simulink model "RoboBoat_Circle_SLAM_v1"  (R2014a)
settings: Solver=FixedStepDiscrete  StartTime=0.0  StopTime=inf  FixedStep=.1  RelTol=1e-3
undefined symbols (not defined in the file): Com1, Com2, Com3, Com4, DiscIntNeverNeededParam, standard
libraries: xpcseriallib x29, slrtlib x5, speedgoatlib_IO102 x5, speedgoatlib x1
(part 1 of 2)
settings Model: BufferReuse=off  Creator=wildcat  LastModifiedBy=wildcat
settings SolverCC: EnableConcurrentExecution=on
settings DataIOCC: SignalLoggingSaveFormat=ModelDataLogs
settings OptimizationCC: BlockReduction=off  OptimizeBlockIOStorage=off  BufferReuse=off  GlobalBufferReuse=off  ExpressionFolding=off  LocalBlockOutputs=off
settings DebuggingCC: UnderspecifiedInitializationDetection=Classic  MultiTaskDSMMsg=warning  StateNameClashWarn=warning
settings HardwareCC: ProdIntDivRoundTo=Zero  ProdEndianess=LittleEndian  ProdHWDeviceType=Generic->32-bit x86 compatible
settings RTWCC: SystemTargetFile=slrt.tlc  TemplateMakefile=slrt_default_tmf  Description=Simulink Real-Time  ProcessScript=slrt_make_rtw_hook  RTWCompilerOptimization=On
settings SimulinkRealTimeCC: GeneratePreprocessorConditionals=Disable all  EnableShiftOperators=on

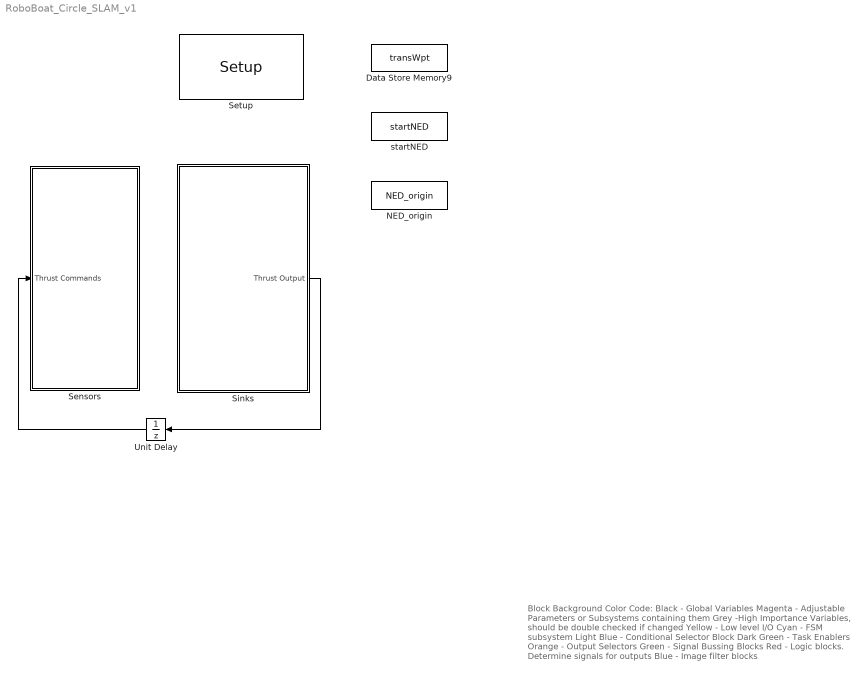
== system RoboBoat_Circle_SLAM_v1 ==
  note: Block Background Color Code:
      | Black - Global Variables
      | Magenta - Adjustable Parameters or Subsystems containing them
      | Grey -High Importance Variables, should be double checked if changed
      | Yellow - Low level I/O
      | Cyan - FSM subsystem
      | Light Blue - Conditional Selector Block
      | Dark Green - Task Enablers
      | Orange - Output Selectors
      | Green - Signal Bussing Blocks
      | Red - Logic blocks. Determine signals for outputs
      | Blue - Image filter blocks
  Data Store Memory9 : DataStoreMemory  DataStoreName=transWpt  ReadBeforeWriteMsg=warning  WriteAfterWriteMsg=warning  WriteAfterReadMsg=warning  InitialValue=[4009.4964500000, 7532.95009000000]
  NED_origin : DataStoreMemory  DataStoreName=NED_origin  ReadBeforeWriteMsg=warning  WriteAfterWriteMsg=warning  WriteAfterReadMsg=warning  InitialValue=[40.1584510000000, -75.5492320000000]  VectorParams1D=off
  Sensors : Subsystem
  Setup : speedgoatlib_IO102/Setup  group=Analog input setup  id=1  range=+-5V  cal=off  pciSlot=-1  adChannelMode=Multiple-channel (enter number of channels below)  adChannel=16  adCoupling=Differential  daChannel=[1,2,3,4]  daReset=[1]  daInitValue=[0]  diChannel=[1,2,3,4,5,6,7,8]  doChannel=[1,2,3,4,5,6,7,8]  doReset=[1]  doInitValue=[0]
  Sinks : Subsystem
  Unit Delay : UnitDelay  SampleTime=-1
  startNED : DataStoreMemory  DataStoreName=startNED  ReadBeforeWriteMsg=warning  WriteAfterWriteMsg=warning  WriteAfterReadMsg=warning  InitialValue=[-10.1298988348139, -7.82721042881905]  VectorParams1D=off
  wires:
  Sinks/1(Thrust Output) -> Unit Delay/1
  Unit Delay/1 -> Sensors/1(Thrust Commands)

== system RoboBoat_Circle_SLAM_v1/Sensors ==
  Thrust Commands : Inport
  1020 Comms : Subsystem  Commented=on
  Baseboard Serial : Subsystem
  Bus Creator : BusCreator  Inputs=3
  IO102 : Subsystem
  data log : Subsystem
  wires:
  Baseboard Serial/1(Serial Inputs) -> Bus Creator/1
  Bus Creator/1 -> data log/1(Sensors signal)  "Serial In"
  IO102/1(IO102 Inputs) -> Bus Creator/2
  Thrust Commands/1 -> Bus Creator/3  "Thrust"

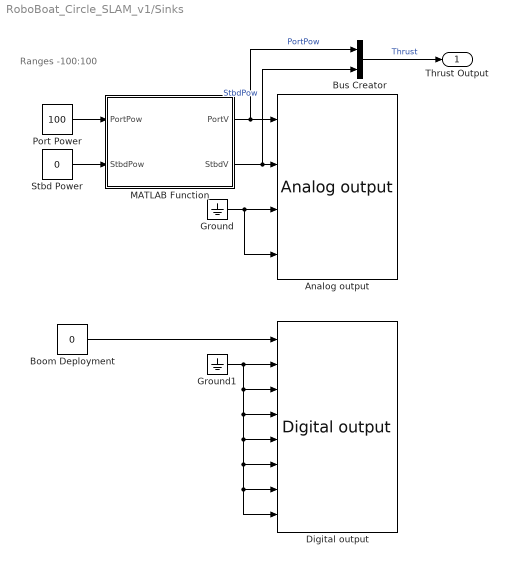
== system RoboBoat_Circle_SLAM_v1/Sinks ==
  note: Ranges -100:100
  Analog output : speedgoatlib_IO102/Analog output  id=1  channels=[1,2,3,4]  range=2  ts=-1  pciSlot=-1
  Boom Deployment : Constant  Value=0
  Bus Creator : BusCreator  Inputs=2
  Digital output : speedgoatlib_IO102/Digital output  id=1  channels=[1,2,3,4,5,6,7,8]  ts=-1  pciSlot=-1
  Ground : Ground
  Ground1 : Ground
  MATLAB Function : MATLAB Function  TreatAsAtomicUnit=on
  Port Power : Constant  Value=100
  Stbd Power : Constant  Value=0
  Thrust Output : Outport
  wires:
  Ground/1 -> Analog output/4, Analog output/3
  Port Power/1 -> MATLAB Function/1(PortPow)
  Stbd Power/1 -> MATLAB Function/2(StbdPow)
  Boom Deployment/1 -> Digital output/1
  Ground1/1 -> Digital output/3, Digital output/4, Digital output/5, Digital output/6, Digital output/7, Digital output/8, Digital output/2
  MATLAB Function/1(PortV) -> Bus Creator/1, Analog output/1  "PortPow"
  MATLAB Function/2(StbdV) -> Bus Creator/2, Analog output/2  "StbdPow"
  Bus Creator/1 -> Thrust Output/1  "Thrust"

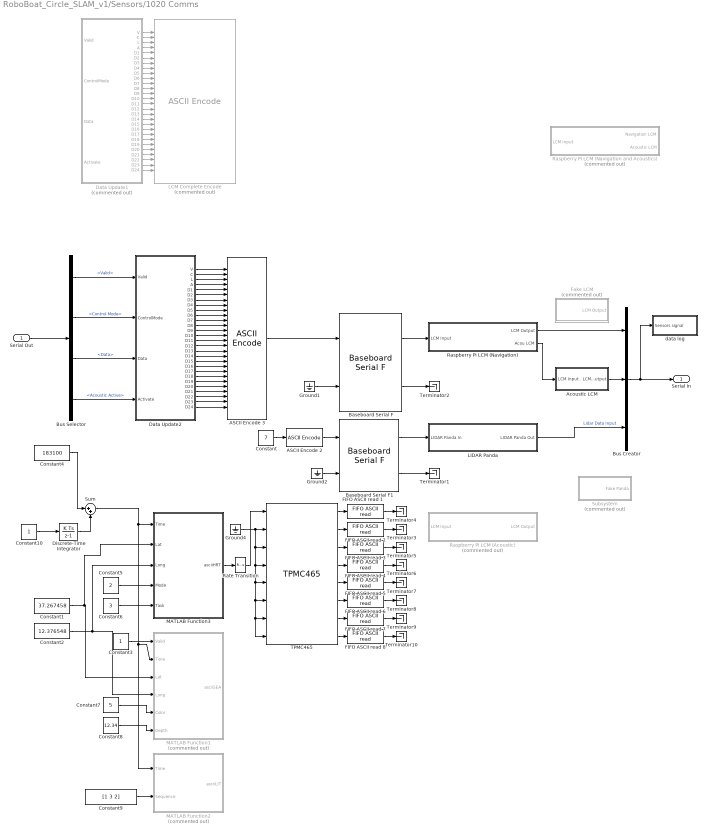
== system RoboBoat_Circle_SLAM_v1/Sensors/1020 Comms ==
  Serial Out : Inport
  " Raspberry Pi LCM (Acoustic)" : Subsystem  Commented=on
  " Raspberry Pi LCM (Navigation and Acoustics)" : Subsystem  Commented=on
  " Raspberry Pi LCM (Navigation)" : Subsystem
  ASCII Encode 2 : xpcseriallib/ASCII Encode   format=SGTask:%d \r\n  nvars=1  maxlength=128  vartypes={ 'double' }
  ASCII Encode 3 : xpcseriallib/ASCII Encode   format="{\"Valid\":%d, \"Mode\":%d, \"Length\":%d, \"Activate\":%d, \"Waypoints\":[%f, %f, %f, %f, %f, %f, %f, %f, %f, %f, %f, %f, %f, %f, %f, %f, %f, %f, %f, %f, %f, %f, %f, %f]} \\r\\n"  nvars=28  maxlength=1000  vartypes={ 'double' }
  Acoustic LCM : Subsystem
  Baseboard Serial F : xpcseriallib/Mainboard/Baseboard Serial F  group=Basic Setup  port=1  irqnum=4  saddr1=0x3f8  saddr2=0x3e8  config=Com1/Com3  baud1=115200  parity1=Even  ndata1=7  nstop1=1  fifomode1=64 deep  rlevel1=1  automode1=on  xmtfifosize1=1024  xmtdatatype1=8 bit uint null terminated  rcvfifosize1=1024  baud2=115200  parity2=Even  ndata2=7  nstop2=1  fifomode2=64 deep  rlevel2=1  automode2=on  xmtfifosize2=1024  xmtdatatype2=8 bit uint null terminated  rcvfifosize2=1024
  Baseboard Serial F1 : xpcseriallib/Mainboard/Baseboard Serial F  group=FIFO Setup  port=1  irqnum=4  saddr1=0x3f8  saddr2=0x3e8  config=Com2/Com4  baud1=115200  parity1=Even  ndata1=7  nstop1=1  fifomode1=64 deep  rlevel1=1  automode1=on  xmtfifosize1=1024  xmtdatatype1=8 bit uint null terminated  rcvfifosize1=1024  baud2=115200  parity2=Even  ndata2=7  nstop2=1  fifomode2=64 deep  rlevel2=1  automode2=on  xmtfifosize2=1024  xmtdatatype2=8 bit uint null terminated  rcvfifosize2=1024
  Bus Creator : BusCreator  Inputs=3
  Bus Selector : BusSelector  OutputSignals=Outputs.Navigation Outputs.Valid,Outputs.Navigation Outputs.Control Mode,Outputs.Navigation Outputs.Data,Outputs.Acoustic Active
  Constant : Constant  Value=7
  Constant1 : Constant  Value=37.267458
  Constant10 : Constant
  Constant2 : Constant  Value=12.376548
  Constant3 : Constant
  Constant4 : Constant  Value=183100
  Constant5 : Constant  Value=2
  Constant6 : Constant  Value=3
  Constant7 : Constant  Value=5
  Constant8 : Constant  Value=12.34
  Constant9 : Constant  Value=[1 3 2]
  Data Update1 : MATLAB Function  Commented=on  TreatAsAtomicUnit=on
  Data Update2 : MATLAB Function  TreatAsAtomicUnit=on
  Discrete-Time Integrator : DiscreteIntegrator  SampleTime=-1  ICPrevOutput=DiscIntNeverNeededParam  ICPrevScaledInput=DiscIntNeverNeededParam
  FIFO ASCII read {1..8} (8 alike) : xpcseriallib/FIFO ASCII read   header={'Deploy:'}  term=[13 10]  hold=Zero output if no new data  enable=off  maxsize=1024  outputtype=8 bit uint null terminated  sampletime=-1
  Fake LCM : Subsystem  Commented=on
  Ground1 : Ground
  Ground2 : Ground
  Ground4 : Ground
  LCM Complete Encode : xpcseriallib/ASCII Encode   Commented=on  format="{\"Valid\":%d, \"Mode\":%d, \"Length\":%d, \"Activate\":%d, \"Waypoints\":[%f, %f, %f, %f, %f, %f, %f, %f, %f, %f, %f, %f, %f, %f, %f, %f, %f, %f, %f, %f, %f, %f, %f, %f]} \\r\\n"  nvars=28  maxlength=1000  vartypes={ 'double' }
  LIDAR Panda : Subsystem
  MATLAB Function1 : MATLAB Function  Commented=on  TreatAsAtomicUnit=on
  MATLAB Function2 : MATLAB Function  Commented=on  TreatAsAtomicUnit=on
  MATLAB Function3 : MATLAB Function  TreatAsAtomicUnit=on
  Rate Transition : RateTransition  Deterministic=off  OutPortSampleTime=1
  Subsystem : Subsystem  Commented=on
  Sum : Sum  Inputs=|++
  TPMC465 : speedgoatlib/IO504/TPMC465  group=Basic Setup  port=2  irqnum=9  slot=-1  transceiver1=RS232 (max 921.6kb/s)  standard1=on  baud1=115200  bauddivisor1=1  sampling1=16x (standard)  prescale1=off  parity1=Even  ndata1=7  nstop1=1  rlevel1=half full (32)  hwmode1=none  swmode1=none  xonchar1=17  xoffchar1=19  rs485auto1=off  rs485delay1=0  xmtfifosize1=1024  xmtdatatype1=8 bit uint null terminated  rcvfifosize1=1024  transceiver2=RS232 (max 921.6kb/s)  standard2=on  baud2=115200  bauddivisor2=1  sampling2=16x (standard)  prescale2=off  parity2=Even  ndata2=7  nstop2=1  rlevel2=half full (32)  hwmode2=none  swmode2=none  xonchar2=17  xoffchar2=19  rs485auto2=off  rs485delay2=0  xmtfifosize2=1024  xmtdatatype2=8 bit uint null terminated  rcvfifosize2=1024  transceiver3=RS232 (max 921.6kb/s)  standard3=on  baud3=115200  bauddivisor3=1  sampling3=16x (standard)  prescale3=off  parity3=Even  ndata3=7  nstop3=1  rlevel3=half full (32)  hwmode3=none  swmode3=none  xonchar3=17  xoffchar3=19  rs485auto3=off  rs485delay3=0  xmtfifosize3=1024  xmtdatatype3=8 bit uint null terminated  rcvfifosize3=1024  transceiver4=RS232 (max 921.6kb/s)  standard4=on  baud4=115200  bauddivisor4=1  sampling4=16x (standard)  prescale4=off  parity4=None  ndata4=8  nstop4=1  rlevel4=half full (32)  hwmode4=none  swmode4=none  xonchar4=17  xoffchar4=19  rs485auto4=off  rs485delay4=0  xmtfifosize4=1024  xmtdatatype4=8 bit uint null terminated  rcvfifosize4=1024  transceiver5=RS232 (max 921.6kb/s)  standard5=on  baud5=115200  bauddivisor5=1  sampling5=16x (standard)  prescale5=off  parity5=None  ndata5=8  nstop5=1  rlevel5=1  hwmode5=none  swmode5=none  xonchar5=17  xoffchar5=19  rs485auto5=off  rs485delay5=0  xmtfifosize5=1024  xmtdatatype5=8 bit uint null terminated  rcvfifosize5=1024  transceiver6=RS232 (max 921.6kb/s)  standard6=on  baud6=115200  bauddivisor6=1  sampling6=16x (standard)  prescale6=off  parity6=None  ndata6=8  nstop6=1  rlevel6=1  hwmode6=none  swmode6=none  xonchar6=17  xoffchar6=19  rs485auto6=off  rs485delay6=0  xmtfifosize6=1024  xmtdatatype6=8 bit uint null terminated  rcvfifosize6=1024  transceiver7=RS232 (max 921.6kb/s)  standard7=on  baud7=115200  bauddivisor7=1  sampling7=16x (standard)  prescale7=off  parity7=None  ndata7=8  nstop7=1  rlevel7=1  hwmode7=none  swmode7=none  xonchar7=17  xoffchar7=19  rs485auto7=off  rs485delay7=0  xmtfifosize7=1024  xmtdatatype7=8 bit uint null terminated  rcvfifosize7=1024  transceiver8=RS232 (max 921.6kb/s)  standard8=on  baud8=115200  bauddivisor8=1  sampling8=16x (standard)  prescale8=off  parity8=None  ndata8=8  nstop8=1  rlevel8=1  hwmode8=none  swmode8=none  xonchar8=17  xoffchar8=19  rs485auto8=off  rs485delay8=0  xmtfifosize8=1024  xmtdatatype8=8 bit uint null terminated  rcvfifosize8=1024
  Terminator{1..10} (10 alike) : Terminator
  data log : Subsystem
  Serial In : Outport
  wires:
  Serial Out/1 -> Bus Selector/1
  Baseboard Serial F/1 -> " Raspberry Pi LCM (Navigation)"/1(LCM Input)
  ASCII Encode 3/1 -> Baseboard Serial F/1
  " Raspberry Pi LCM (Navigation)"/1(LCM Output) -> Bus Creator/1
  Bus Selector/1 -> Data Update2/1(Valid)  "<Valid>"
  Bus Selector/2 -> Data Update2/2(ControlMode)  "<Control Mode>"
  Bus Selector/3 -> Data Update2/3(Data)  "<Data>"
  Acoustic LCM/1(LCM Output) -> Bus Creator/2
  Baseboard Serial F/2 -> Terminator2/1
  Ground1/1 -> Baseboard Serial F/2
  LIDAR Panda/1(LIDAR Panda Out) -> Bus Creator/3  "Lidar Data Input"
  Bus Creator/1 -> Serial In/1, data log/1(Sensors signal)
  Data Update1/1(V) -> LCM Complete Encode/1
  Data Update1/2(C) -> LCM Complete Encode/2
  Data Update1/6(D2) -> LCM Complete Encode/6
  Data Update1/7(D3) -> LCM Complete Encode/7
  Data Update1/8(D4) -> LCM Complete Encode/8
  Data Update1/5(D1) -> LCM Complete Encode/5
  Data Update1/9(D5) -> LCM Complete Encode/9
  Data Update1/10(D6) -> LCM Complete Encode/10
  Data Update1/11(D7) -> LCM Complete Encode/11
  Data Update1/12(D8) -> LCM Complete Encode/12
  Data Update1/13(D9) -> LCM Complete Encode/13
  Data Update1/18(D14) -> LCM Complete Encode/18
  Data Update1/15(D11) -> LCM Complete Encode/15
  Data Update1/20(D16) -> LCM Complete Encode/20
  Data Update1/21(D17) -> LCM Complete Encode/21
  Data Update1/19(D15) -> LCM Complete Encode/19
  Data Update1/14(D10) -> LCM Complete Encode/14
  Data Update1/16(D12) -> LCM Complete Encode/16
  Data Update1/22(D18) -> LCM Complete Encode/22
  Data Update1/23(D19) -> LCM Complete Encode/23
  Data Update1/24(D20) -> LCM Complete Encode/24
  Data Update1/25(D21) -> LCM Complete Encode/25
  Data Update1/27(D23) -> LCM Complete Encode/27
  Data Update1/26(D22) -> LCM Complete Encode/26
  Data Update1/28(D24) -> LCM Complete Encode/28
  Data Update1/3(L) -> LCM Complete Encode/3
  Data Update1/4(A) -> LCM Complete Encode/4
  Data Update1/17(D13) -> LCM Complete Encode/17
  " Raspberry Pi LCM (Navigation)"/2(Acou LCM) -> Acoustic LCM/1(LCM Input)
  Data Update2/21(D17) -> ASCII Encode 3/21
  Data Update2/20(D16) -> ASCII Encode 3/20
  Data Update2/19(D15) -> ASCII Encode 3/19
  Data Update2/4(A) -> ASCII Encode 3/4
  Data Update2/2(C) -> ASCII Encode 3/2
  Data Update2/18(D14) -> ASCII Encode 3/18
  Data Update2/16(D12) -> ASCII Encode 3/16
  Data Update2/7(D3) -> ASCII Encode 3/7
  Data Update2/6(D2) -> ASCII Encode 3/6
  Data Update2/5(D1) -> ASCII Encode 3/5
  Data Update2/17(D13) -> ASCII Encode 3/17
  Data Update2/9(D5) -> ASCII Encode 3/9
  Data Update2/10(D6) -> ASCII Encode 3/10
  Data Update2/24(D20) -> ASCII Encode 3/24
  Data Update2/23(D19) -> ASCII Encode 3/23
  Data Update2/28(D24) -> ASCII Encode 3/28
  Data Update2/26(D22) -> ASCII Encode 3/26
  Data Update2/25(D21) -> ASCII Encode 3/25
  Data Update2/3(L) -> ASCII Encode 3/3
  Data Update2/27(D23) -> ASCII Encode 3/27
  Data Update2/8(D4) -> ASCII Encode 3/8
  Data Update2/11(D7) -> ASCII Encode 3/11
  Data Update2/13(D9) -> ASCII Encode 3/13
  Data Update2/12(D8) -> ASCII Encode 3/12
  Data Update2/14(D10) -> ASCII Encode 3/14
  Data Update2/22(D18) -> ASCII Encode 3/22
  Data Update2/15(D11) -> ASCII Encode 3/15
  Bus Selector/4 -> Data Update2/4(Activate)  "<Acoustic Active>"
  Data Update2/1(V) -> ASCII Encode 3/1
  Constant9/1 -> MATLAB Function2/2(Sequence)
  Constant7/1 -> MATLAB Function1/5(Color)
  Constant8/1 -> MATLAB Function1/6(Depth)
  Constant5/1 -> MATLAB Function3/4(Mode)
  Constant6/1 -> MATLAB Function3/5(Task)
  Sum/1 -> MATLAB Function3/1(Time), MATLAB Function2/1(Time), MATLAB Function1/2(Time)
  Constant2/1 -> MATLAB Function3/3(Long), MATLAB Function1/4(Long)
  Constant1/1 -> MATLAB Function3/2(Lat), MATLAB Function1/3(Lat)
  Ground4/1 -> TPMC465/2, TPMC465/3, TPMC465/4, TPMC465/8, TPMC465/7, TPMC465/6, TPMC465/5
  TPMC465/1 -> FIFO ASCII read 1/1
  FIFO ASCII read 1/1 -> Terminator4/1
  FIFO ASCII read 2/1 -> Terminator3/1
  FIFO ASCII read 3/1 -> Terminator5/1
  FIFO ASCII read 4/1 -> Terminator6/1
  FIFO ASCII read 5/1 -> Terminator7/1
  FIFO ASCII read 6/1 -> Terminator8/1
  FIFO ASCII read 7/1 -> Terminator9/1
  FIFO ASCII read 8/1 -> Terminator10/1
  TPMC465/2 -> FIFO ASCII read 2/1
  TPMC465/3 -> FIFO ASCII read 3/1
  TPMC465/4 -> FIFO ASCII read 4/1
  TPMC465/5 -> FIFO ASCII read 5/1
  TPMC465/6 -> FIFO ASCII read 6/1
  TPMC465/7 -> FIFO ASCII read 7/1
  TPMC465/8 -> FIFO ASCII read 8/1
  Rate Transition/1 -> TPMC465/1
  Constant3/1 -> MATLAB Function1/1(Valid)
  MATLAB Function3/1(asciiHRT) -> Rate Transition/1
  Constant4/1 -> Sum/1
  Discrete-Time Integrator/1 -> Sum/2
  Constant10/1 -> Discrete-Time Integrator/1
  Baseboard Serial F1/1 -> LIDAR Panda/1(LIDAR Panda In)
  Ground2/1 -> Baseboard Serial F1/2
  Baseboard Serial F1/2 -> Terminator1/1
  ASCII Encode 2/1 -> Baseboard Serial F1/1
  Constant/1 -> ASCII Encode 2/1

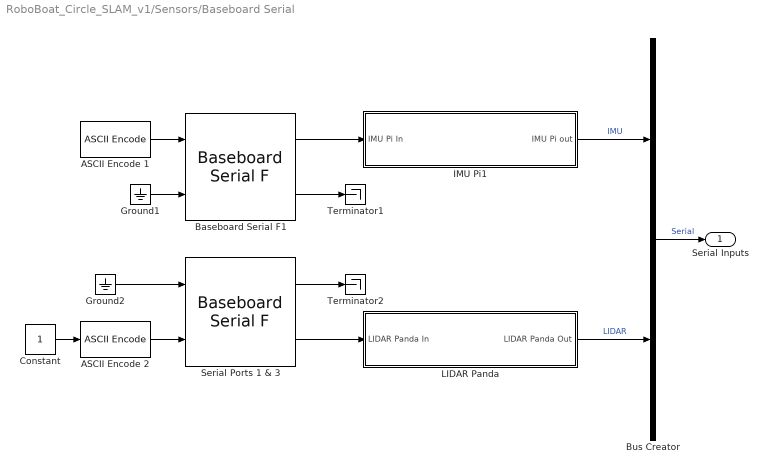
== system RoboBoat_Circle_SLAM_v1/Sensors/Baseboard Serial ==
  ASCII Encode 1 : xpcseriallib/ASCII Encode   format=SGB \r\n  nvars=0  maxlength=128  vartypes={ 'double' }
  ASCII Encode 2 : xpcseriallib/ASCII Encode   format=SGTask:%d \r\n  nvars=1  maxlength=128  vartypes={ 'double' }
  Baseboard Serial F1 : xpcseriallib/Mainboard/Baseboard Serial F  group=Basic Setup  port=1  irqnum=4  saddr1=0x3f8  saddr2=0x3e8  config=Com2/Com4  baud1=115200  parity1=Even  ndata1=7  nstop1=1  fifomode1=64 deep  rlevel1=1  automode1=on  xmtfifosize1=1024  xmtdatatype1=8 bit uint null terminated  rcvfifosize1=1024  baud2=115200  parity2=Even  ndata2=7  nstop2=1  fifomode2=64 deep  rlevel2=1  automode2=on  xmtfifosize2=1024  xmtdatatype2=8 bit uint null terminated  rcvfifosize2=1024
  Bus Creator : BusCreator  Inputs=2
  Constant : Constant
  Ground1 : Ground
  Ground2 : Ground
  IMU Pi1 : Subsystem
  LIDAR Panda : Subsystem
  Serial Ports 1 & 3 : xpcseriallib/Mainboard/Baseboard Serial F  group=Basic Setup  port=2  irqnum=4  saddr1=0x3f8  saddr2=0x3e8  config=Com1/Com3  baud1=115200  parity1=Even  ndata1=7  nstop1=1  fifomode1=64 deep  rlevel1=1  automode1=on  xmtfifosize1=1024  xmtdatatype1=8 bit uint null terminated  rcvfifosize1=1024  baud2=115200  parity2=Even  ndata2=7  nstop2=1  fifomode2=64 deep  rlevel2=1  automode2=on  xmtfifosize2=1024  xmtdatatype2=8 bit uint null terminated  rcvfifosize2=1024
  Terminator1 : Terminator
  Terminator2 : Terminator
  Serial Inputs : Outport
  wires:
  Baseboard Serial F1/1 -> IMU Pi1/1(IMU Pi In)
  Ground1/1 -> Baseboard Serial F1/2
  Baseboard Serial F1/2 -> Terminator1/1
  Ground2/1 -> Serial Ports 1 & 3/1
  Serial Ports 1 & 3/2 -> LIDAR Panda/1(LIDAR Panda In)
  Constant/1 -> ASCII Encode 2/1
  ASCII Encode 2/1 -> Serial Ports 1 & 3/2
  Serial Ports 1 & 3/1 -> Terminator2/1
  LIDAR Panda/1(LIDAR Panda Out) -> Bus Creator/2  "LIDAR"
  Bus Creator/1 -> Serial Inputs/1  "Serial"
  IMU Pi1/1(IMU Pi out) -> Bus Creator/1  "IMU"
  ASCII Encode 1/1 -> Baseboard Serial F1/1

== system RoboBoat_Circle_SLAM_v1/Sensors/IO102 ==
  Analog In : Subsystem
  Bus Creator : BusCreator  Inputs=2
  Digital In : Subsystem
  IO102 Inputs : Outport
  wires:
  Digital In/1(Digital In) -> Bus Creator/1  "Digital"
  Analog In/1(Analog In) -> Bus Creator/2  "Analog"
  Bus Creator/1 -> IO102 Inputs/1  "IO102"

== system RoboBoat_Circle_SLAM_v1/Sensors/data log ==
  Sensors signal : Inport
  Bus to Vector : BusToVector
  Scope 2 : slrtlib/Displays and Logging/Scope   scopeno=2  scopetype=File  autostart=on  viewmode=Graphical redraw  formatstr='%15.6f'  grid=on  ylimits=[0,0]  nosamples=250  noprepostsamples=0  interleave=1  triggermode=FreeRun  triggersignal=1  trigsignalfromport=off  triggerlevel=0.0  triggerslope=Either  triggerscope=1  triggersample=0  filename=SEN_<%%%>.dat  mode=Commit  writesize=512  autorestart=on  dynamicfilemode=on  maxwritefilesize=512*6000^2
  wires:
  Bus to Vector/1 -> Scope 2/1
  Sensors signal/1 -> Bus to Vector/1

== system RoboBoat_Circle_SLAM_v1/Sensors/1020 Comms/ Raspberry Pi LCM (Acoustic) ==
  LCM Input : Inport
  ASCII Decode 6 : xpcseriallib/ASCII Decode   format=Deploy:%1u, Elapsed:%g, Bearing1:%g Bearing2:%g \r\n  nvars=4  vartypes={}
  Bus Creator : BusCreator  Inputs=2
  Bus Creator1 : BusCreator  Inputs=3
  FIFO ASCII read 1 : xpcseriallib/FIFO ASCII read   header={'Deploy:'}  term=[13 10]  hold=Zero output if no new data  enable=off  maxsize=1024  outputtype=8 bit uint null terminated  sampletime=-1
  LCM Output : Outport
  wires:
  LCM Input/1 -> FIFO ASCII read 1/1
  FIFO ASCII read 1/1 -> ASCII Decode 6/1
  ASCII Decode 6/3 -> Bus Creator/1  "Horizontal Bearing"
  ASCII Decode 6/4 -> Bus Creator/2  "Vertical Bearing"
  Bus Creator/1 -> Bus Creator1/3  "Bearings"
  ASCII Decode 6/2 -> Bus Creator1/2  "Elapsed Time"
  ASCII Decode 6/1 -> Bus Creator1/1  "Deployed"
  Bus Creator1/1 -> LCM Output/1  "Acoustic Message"

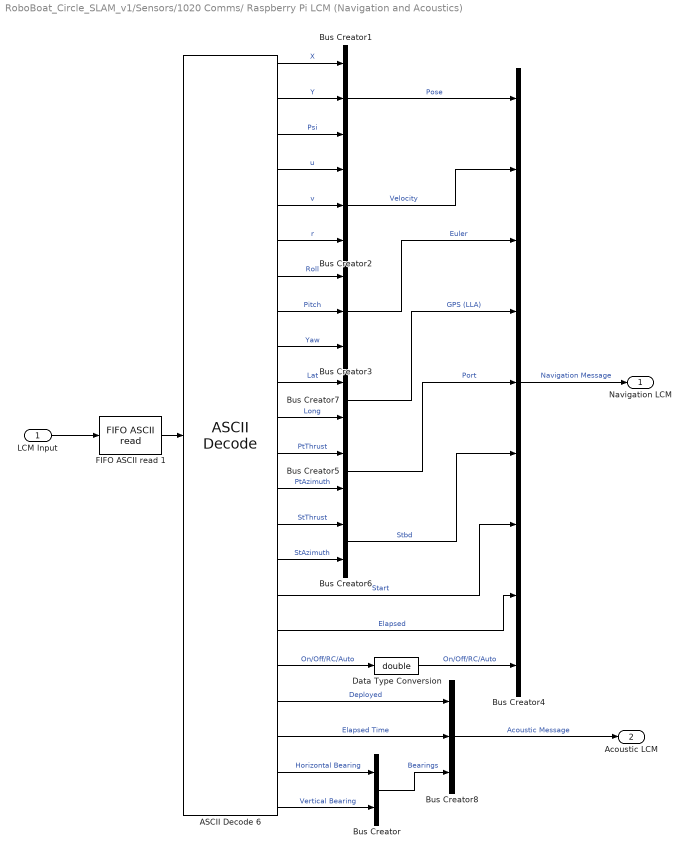
== system RoboBoat_Circle_SLAM_v1/Sensors/1020 Comms/ Raspberry Pi LCM (Navigation and Acoustics) ==
  LCM Input : Inport
  ASCII Decode 6 : xpcseriallib/ASCII Decode   format=P1:%f P2:%f P3:%f V1:%f V2:%f V3:%f E1:%f E2:%f E3:%f Pt1:%f Pt2:%f St1:%f St2:%f Start:%f Elapsed:%f RC:%d Deploy:%u, Elapsed:%g, Bearing1:%g Bearing2:%g \r\n  nvars=22  vartypes={}
  Bus Creator{,5..7} (4 alike) : BusCreator  Inputs=2
  Bus Creator{1..3,8} (4 alike) : BusCreator  Inputs=3
  Bus Creator4 : BusCreator  Inputs=9
  Data Type Conversion : DataTypeConversion  OutDataTypeStr=double
  FIFO ASCII read 1 : xpcseriallib/FIFO ASCII read   header={'P1:'}  term=[13 10]  hold=Zero output if no new data  enable=off  maxsize=2048  outputtype=8 bit uint null terminated  sampletime=-1
  Navigation LCM : Outport
  Acoustic LCM : Outport  Port=2
  wires:
  LCM Input/1 -> FIFO ASCII read 1/1
  FIFO ASCII read 1/1 -> ASCII Decode 6/1
  Bus Creator4/1 -> Navigation LCM/1  "Navigation Message"
  ASCII Decode 6/1 -> Bus Creator1/1  "X"
  ASCII Decode 6/2 -> Bus Creator1/2  "Y"
  ASCII Decode 6/3 -> Bus Creator1/3  "Psi"
  Bus Creator1/1 -> Bus Creator4/1  "Pose"
  ASCII Decode 6/4 -> Bus Creator2/1  "u"
  ASCII Decode 6/5 -> Bus Creator2/2  "v"
  Bus Creator2/1 -> Bus Creator4/2  "Velocity"
  ASCII Decode 6/7 -> Bus Creator3/1  "Roll"
  ASCII Decode 6/8 -> Bus Creator3/2  "Pitch"
  ASCII Decode 6/9 -> Bus Creator3/3  "Yaw"
  Bus Creator3/1 -> Bus Creator4/3  "Euler"
  Bus Creator5/1 -> Bus Creator4/5  "Port"
  Bus Creator6/1 -> Bus Creator4/6  "Stbd"
  ASCII Decode 6/14 -> Bus Creator6/1  "StThrust"
  ASCII Decode 6/15 -> Bus Creator6/2  "StAzimuth"
  ASCII Decode 6/12 -> Bus Creator5/1  "PtThrust"
  ASCII Decode 6/13 -> Bus Creator5/2  "PtAzimuth"
  ASCII Decode 6/16 -> Bus Creator4/7  "Start"
  ASCII Decode 6/17 -> Bus Creator4/8  "Elapsed"
  ASCII Decode 6/18 -> Data Type Conversion/1  "On/Off/RC/Auto"
  Data Type Conversion/1 -> Bus Creator4/9  "On/Off/RC/Auto"
  ASCII Decode 6/6 -> Bus Creator2/3  "r"
  ASCII Decode 6/10 -> Bus Creator7/1  "Lat"
  ASCII Decode 6/11 -> Bus Creator7/2  "Long"
  Bus Creator7/1 -> Bus Creator4/4  "GPS (LLA)"
  ASCII Decode 6/21 -> Bus Creator/1  "Horizontal Bearing"
  ASCII Decode 6/22 -> Bus Creator/2  "Vertical Bearing"
  Bus Creator/1 -> Bus Creator8/3  "Bearings"
  ASCII Decode 6/20 -> Bus Creator8/2  "Elapsed Time"
  ASCII Decode 6/19 -> Bus Creator8/1  "Deployed"
  Bus Creator8/1 -> Acoustic LCM/1  "Acoustic Message"

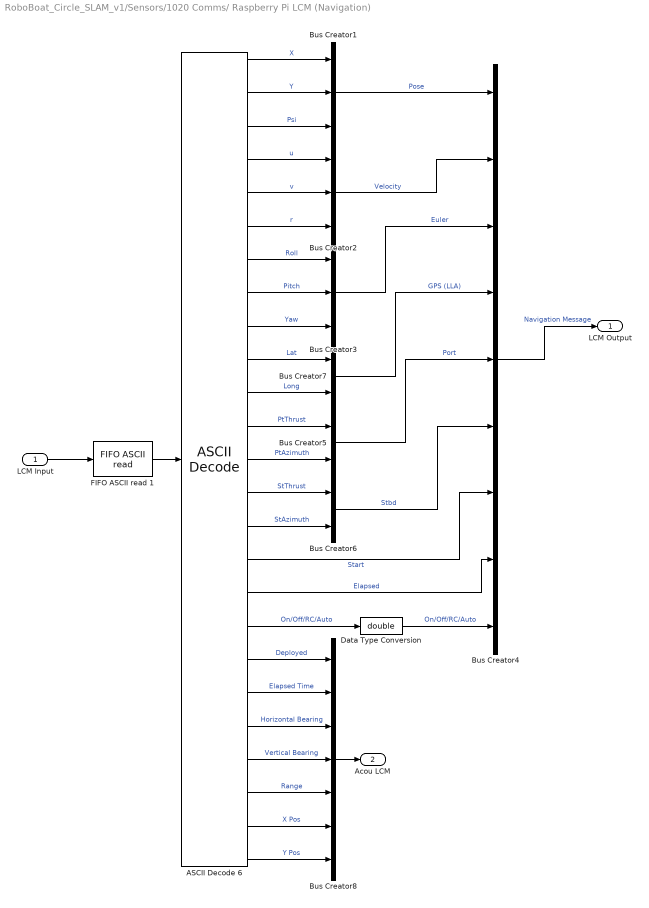
== system RoboBoat_Circle_SLAM_v1/Sensors/1020 Comms/ Raspberry Pi LCM (Navigation) ==
  LCM Input : Inport
  ASCII Decode 6 : xpcseriallib/ASCII Decode   format=P1:%f P2:%f P3:%f V1:%f V2:%f V3:%f E1:%f E2:%f E3:%f Lat:%f Long:%f Pt1:%f Pt2:%f St1:%f St2:%f Start:%f Elapsed:%f RC:%d Deploy:%u Elapsed:%f Bearing1:%f Bearing2:%f Range:%f X_Pos:%f Y_Pos:%f \r\n  nvars=25  vartypes={}
  Bus Creator1 : BusCreator  Inputs=3
  Bus Creator2 : BusCreator  Inputs=3
  Bus Creator3 : BusCreator  Inputs=3
  Bus Creator4 : BusCreator  Inputs=9
  Bus Creator5 : BusCreator  Inputs=2
  Bus Creator6 : BusCreator  Inputs=2
  Bus Creator7 : BusCreator  Inputs=2
  Bus Creator8 : BusCreator  Inputs=7
  Data Type Conversion : DataTypeConversion  OutDataTypeStr=double
  FIFO ASCII read 1 : xpcseriallib/FIFO ASCII read   header={'P1:'}  term=[13 10]  hold=Zero output if no new data  enable=off  maxsize=2000  outputtype=8 bit uint null terminated  sampletime=-1
  LCM Output : Outport
  Acou LCM : Outport  Port=2
  wires:
  LCM Input/1 -> FIFO ASCII read 1/1
  FIFO ASCII read 1/1 -> ASCII Decode 6/1
  Bus Creator4/1 -> LCM Output/1  "Navigation Message"
  ASCII Decode 6/1 -> Bus Creator1/1  "X"
  ASCII Decode 6/2 -> Bus Creator1/2  "Y"
  ASCII Decode 6/3 -> Bus Creator1/3  "Psi"
  Bus Creator1/1 -> Bus Creator4/1  "Pose"
  ASCII Decode 6/4 -> Bus Creator2/1  "u"
  ASCII Decode 6/5 -> Bus Creator2/2  "v"
  Bus Creator2/1 -> Bus Creator4/2  "Velocity"
  ASCII Decode 6/7 -> Bus Creator3/1  "Roll"
  ASCII Decode 6/8 -> Bus Creator3/2  "Pitch"
  ASCII Decode 6/9 -> Bus Creator3/3  "Yaw"
  Bus Creator3/1 -> Bus Creator4/3  "Euler"
  Bus Creator5/1 -> Bus Creator4/5  "Port"
  Bus Creator6/1 -> Bus Creator4/6  "Stbd"
  ASCII Decode 6/14 -> Bus Creator6/1  "StThrust"
  ASCII Decode 6/15 -> Bus Creator6/2  "StAzimuth"
  ASCII Decode 6/12 -> Bus Creator5/1  "PtThrust"
  ASCII Decode 6/13 -> Bus Creator5/2  "PtAzimuth"
  ASCII Decode 6/16 -> Bus Creator4/7  "Start"
  ASCII Decode 6/17 -> Bus Creator4/8  "Elapsed"
  ASCII Decode 6/18 -> Data Type Conversion/1  "On/Off/RC/Auto"
  Data Type Conversion/1 -> Bus Creator4/9  "On/Off/RC/Auto"
  ASCII Decode 6/6 -> Bus Creator2/3  "r"
  ASCII Decode 6/10 -> Bus Creator7/1  "Lat"
  ASCII Decode 6/11 -> Bus Creator7/2  "Long"
  Bus Creator7/1 -> Bus Creator4/4  "GPS (LLA)"
  ASCII Decode 6/19 -> Bus Creator8/1  "Deployed"
  ASCII Decode 6/20 -> Bus Creator8/2  "Elapsed Time"
  ASCII Decode 6/21 -> Bus Creator8/3  "Horizontal Bearing"
  ASCII Decode 6/22 -> Bus Creator8/4  "Vertical Bearing"
  ASCII Decode 6/23 -> Bus Creator8/5  "Range"
  ASCII Decode 6/24 -> Bus Creator8/6  "X Pos"
  ASCII Decode 6/25 -> Bus Creator8/7  "Y Pos"
  Bus Creator8/1 -> Acou LCM/1

== system RoboBoat_Circle_SLAM_v1/Sensors/1020 Comms/Acoustic LCM ==
  LCM Input : Inport
  Bus Creator : BusCreator  Inputs=2
  Bus Creator1 : BusCreator
  Bus Creator2 : BusCreator  Inputs=3
  Bus Selector : BusSelector  OutputSignals=Deployed,Elapsed Time,Horizontal Bearing,Vertical Bearing,Range,X Pos,Y Pos
  LCM Output : Outport
  wires:
  Bus Selector/3 -> Bus Creator/1  "<Horizontal Bearing>"
  Bus Selector/4 -> Bus Creator/2  "<Vertical Bearing>"
  Bus Creator/1 -> Bus Creator1/3  "Bearings"
  Bus Selector/2 -> Bus Creator1/2  "<Elapsed Time>"
  Bus Selector/1 -> Bus Creator1/1  "<Deployed>"
  Bus Creator1/1 -> LCM Output/1  "Acoustic Message"
  LCM Input/1 -> Bus Selector/1
  Bus Selector/5 -> Bus Creator2/1  "<Range>"
  Bus Selector/6 -> Bus Creator2/2  "<X Pos>"
  Bus Selector/7 -> Bus Creator2/3  "<Y Pos>"
  Bus Creator2/1 -> Bus Creator1/4  "Pose Estimate"

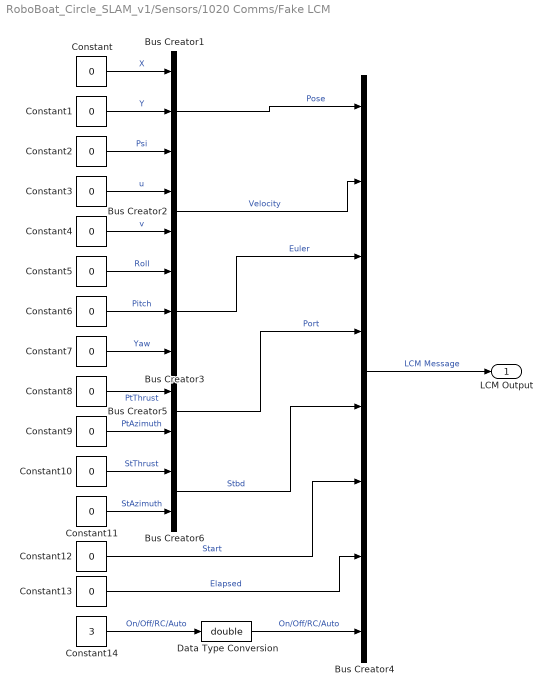
== system RoboBoat_Circle_SLAM_v1/Sensors/1020 Comms/Fake LCM ==
  Bus Creator1 : BusCreator  Inputs=3
  Bus Creator2 : BusCreator  Inputs=2
  Bus Creator3 : BusCreator  Inputs=3
  Bus Creator4 : BusCreator  Inputs=8
  Bus Creator5 : BusCreator  Inputs=2
  Bus Creator6 : BusCreator  Inputs=2
  Constant{,1..13} (14 alike) : Constant  Value=0
  Constant14 : Constant  Value=3
  Data Type Conversion : DataTypeConversion  OutDataTypeStr=double
  LCM Output : Outport
  wires:
  Bus Creator4/1 -> LCM Output/1  "LCM Message"
  Constant/1 -> Bus Creator1/1  "X"
  Constant1/1 -> Bus Creator1/2  "Y"
  Constant2/1 -> Bus Creator1/3  "Psi"
  Bus Creator1/1 -> Bus Creator4/1  "Pose"
  Constant3/1 -> Bus Creator2/1  "u"
  Constant4/1 -> Bus Creator2/2  "v"
  Bus Creator2/1 -> Bus Creator4/2  "Velocity"
  Constant5/1 -> Bus Creator3/1  "Roll"
  Constant6/1 -> Bus Creator3/2  "Pitch"
  Constant7/1 -> Bus Creator3/3  "Yaw"
  Bus Creator3/1 -> Bus Creator4/3  "Euler"
  Bus Creator5/1 -> Bus Creator4/4  "Port"
  Bus Creator6/1 -> Bus Creator4/5  "Stbd"
  Constant10/1 -> Bus Creator6/1  "StThrust"
  Constant11/1 -> Bus Creator6/2  "StAzimuth"
  Constant8/1 -> Bus Creator5/1  "PtThrust"
  Constant9/1 -> Bus Creator5/2  "PtAzimuth"
  Constant12/1 -> Bus Creator4/6  "Start"
  Constant13/1 -> Bus Creator4/7  "Elapsed"
  Constant14/1 -> Data Type Conversion/1  "On/Off/RC/Auto"
  Data Type Conversion/1 -> Bus Creator4/8  "On/Off/RC/Auto"

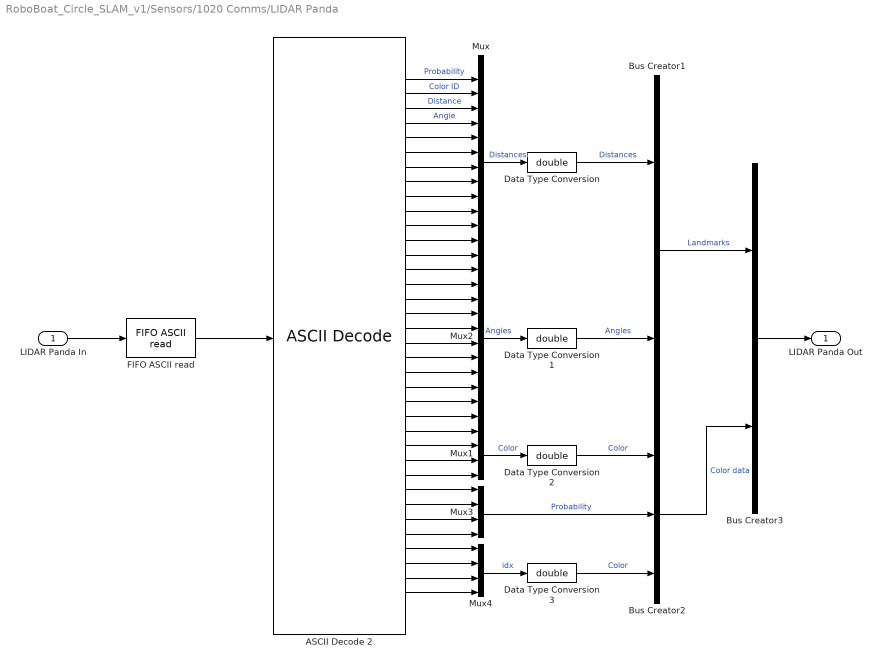
== system RoboBoat_Circle_SLAM_v1/Sensors/1020 Comms/LIDAR Panda ==
  LIDAR Panda In : Inport
  ASCII Decode 2 : xpcseriallib/ASCII Decode   format=A:%d B:%d C:%d E:%d F:%d G:%d H:%d I:%d J:%d K:%d L:%d M:%d N:%d O:%d P:%d Q:%d R:%d S:%d T:%d U:%d V:%d W:%d X:%d C1:%d C2:%d C3:%d C4:%d P1:%f P2:%f P3:%f P4:%f I1:%d I2:%d I3:%d I4:%d \r\n  nvars=36  vartypes={}
  Bus Creator1 : BusCreator  Inputs=2
  Bus Creator2 : BusCreator  Inputs=3
  Bus Creator3 : BusCreator  Inputs=2
  Data Type Conversion{,1..3} (4 alike) : DataTypeConversion  OutDataTypeStr=double
  "FIFO ASCII read " : xpcseriallib/FIFO ASCII read   header={'A:'}  term=[13 10]  hold=Zero output if no new data  enable=off  maxsize=1024  outputtype=8 bit uint null terminated  sampletime=-1
  Mux : Mux  Inputs=12
  Mux1 : Mux
  Mux2 : Mux  Inputs=12
  Mux3 : Mux
  Mux4 : Mux
  LIDAR Panda Out : Outport
  wires:
  LIDAR Panda In/1 -> "FIFO ASCII read "/1
  "FIFO ASCII read "/1 -> ASCII Decode 2/1
  ASCII Decode 2/3 -> Mux/3  "Distance"
  ASCII Decode 2/2 -> Mux/2  "Color ID"
  ASCII Decode 2/4 -> Mux/4  "Angle"
  ASCII Decode 2/1 -> Mux/1  "Probability"
  ASCII Decode 2/7 -> Mux/7
  ASCII Decode 2/10 -> Mux/10
  ASCII Decode 2/11 -> Mux/11
  ASCII Decode 2/6 -> Mux/6
  ASCII Decode 2/8 -> Mux/8
  ASCII Decode 2/9 -> Mux/9
  ASCII Decode 2/12 -> Mux/12
  ASCII Decode 2/5 -> Mux/5
  ASCII Decode 2/13 -> Mux2/1
  ASCII Decode 2/15 -> Mux2/3
  ASCII Decode 2/22 -> Mux2/10
  ASCII Decode 2/23 -> Mux2/11
  ASCII Decode 2/17 -> Mux2/5
  ASCII Decode 2/18 -> Mux2/6
  ASCII Decode 2/14 -> Mux2/2
  ASCII Decode 2/24 -> Mux2/12
  ASCII Decode 2/20 -> Mux2/8
  ASCII Decode 2/19 -> Mux2/7
  ASCII Decode 2/21 -> Mux2/9
  ASCII Decode 2/16 -> Mux2/4
  ASCII Decode 2/25 -> Mux1/1
  ASCII Decode 2/28 -> Mux1/4
  ASCII Decode 2/26 -> Mux1/2
  ASCII Decode 2/27 -> Mux1/3
  ASCII Decode 2/30 -> Mux3/2
  ASCII Decode 2/31 -> Mux3/3
  ASCII Decode 2/32 -> Mux3/4
  ASCII Decode 2/29 -> Mux3/1
  ASCII Decode 2/36 -> Mux4/4
  ASCII Decode 2/34 -> Mux4/2
  ASCII Decode 2/35 -> Mux4/3
  ASCII Decode 2/33 -> Mux4/1
  Mux/1 -> Data Type Conversion/1  "Distances"
  Mux2/1 -> Data Type Conversion1/1  "Angles"
  Mux1/1 -> Data Type Conversion2/1  "Color"
  Mux3/1 -> Bus Creator2/2  "Probability"
  Mux4/1 -> Data Type Conversion3/1  "idx"
  Bus Creator1/1 -> Bus Creator3/1  "Landmarks"
  Bus Creator2/1 -> Bus Creator3/2  "Color data"
  Bus Creator3/1 -> LIDAR Panda Out/1
  Data Type Conversion/1 -> Bus Creator1/1  "Distances"
  Data Type Conversion1/1 -> Bus Creator1/2  "Angles"
  Data Type Conversion2/1 -> Bus Creator2/1  "Color"
  Data Type Conversion3/1 -> Bus Creator2/3  "Color"

== system RoboBoat_Circle_SLAM_v1/Sensors/1020 Comms/Subsystem ==
  Bus Creator : BusCreator  Inputs=3
  Bus Creator1 : BusCreator  Inputs=2
  Bus Creator2 : BusCreator  Inputs=2
  Constant : Constant  Value=zeros(12,1)
  Constant1 : Constant  Value=zeros(12,1)
  Constant2 : Constant  Value=zeros(4,1)
  Constant3 : Constant  Value=zeros(4,1)
  Constant4 : Constant  Value=zeros(4,1)
  Fake Panda : Outport
  wires:
  Constant/1 -> Bus Creator1/1  "Distances"
  Constant1/1 -> Bus Creator1/2  "Angles"
  Constant2/1 -> Bus Creator/1  "Color"
  Constant3/1 -> Bus Creator/2  "Probability"
  Constant4/1 -> Bus Creator/3  "idx"
  Bus Creator1/1 -> Bus Creator2/1  "Landmarks"
  Bus Creator/1 -> Bus Creator2/2  "Color data"
  Bus Creator2/1 -> Fake Panda/1  "Lidar Data Input"

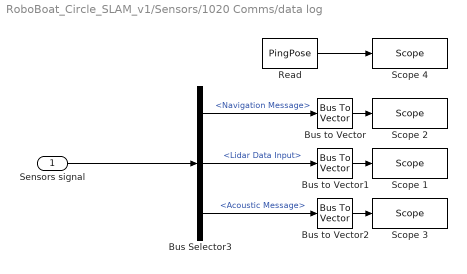
== system RoboBoat_Circle_SLAM_v1/Sensors/1020 Comms/data log ==
  Sensors signal : Inport
  Bus Selector3 : BusSelector  OutputSignals=Navigation Message,Lidar Data Input,Acoustic Message
  Bus to Vector : BusToVector
  Bus to Vector1 : BusToVector
  Bus to Vector2 : BusToVector
  Read : DataStoreRead  DataStoreName=PingPose
  Scope 1 : slrtlib/Displays and Logging/Scope   scopeno=3  scopetype=File  autostart=on  viewmode=Graphical redraw  formatstr='%15.6f'  grid=on  ylimits=[0,0]  nosamples=28800  noprepostsamples=0  interleave=1  triggermode=FreeRun  triggersignal=1  trigsignalfromport=off  triggerlevel=0.0  triggerslope=Either  triggerscope=1  triggersample=0  filename=LM1_<%%%>.dat  mode=Lazy  writesize=5120  autorestart=on  dynamicfilemode=on  maxwritefilesize=512*1024^2
  Scope 2 : slrtlib/Displays and Logging/Scope   scopeno=1  scopetype=File  autostart=on  viewmode=Graphical redraw  formatstr='%15.6f'  grid=on  ylimits=[0,0]  nosamples=28800  noprepostsamples=0  interleave=1  triggermode=FreeRun  triggersignal=1  trigsignalfromport=off  triggerlevel=0.0  triggerslope=Either  triggerscope=1  triggersample=0  filename=NAV1_<%%%>.dat  mode=Lazy  writesize=5120  autorestart=on  dynamicfilemode=on  maxwritefilesize=512*1024^2
  Scope 3 : slrtlib/Displays and Logging/Scope   scopeno=2  scopetype=File  autostart=on  viewmode=Graphical redraw  formatstr='%15.6f'  grid=on  ylimits=[0,0]  nosamples=28800  noprepostsamples=0  interleave=1  triggermode=FreeRun  triggersignal=1  trigsignalfromport=off  triggerlevel=0.0  triggerslope=Either  triggerscope=1  triggersample=0  filename=ACO1_<%%%>.dat  mode=Lazy  writesize=5120  autorestart=on  dynamicfilemode=on  maxwritefilesize=512*1024^2
  Scope 4 : slrtlib/Displays and Logging/Scope   scopeno=4  scopetype=File  autostart=on  viewmode=Graphical redraw  formatstr='%15.6f'  grid=on  ylimits=[0,0]  nosamples=28800  noprepostsamples=0  interleave=1  triggermode=FreeRun  triggersignal=1  trigsignalfromport=off  triggerlevel=0.0  triggerslope=Either  triggerscope=1  triggersample=0  filename=pPos_<%%%>.dat  mode=Lazy  writesize=5120  autorestart=on  dynamicfilemode=on  maxwritefilesize=512*1024^2
  wires:
  Sensors signal/1 -> Bus Selector3/1
  Bus to Vector/1 -> Scope 2/1
  Bus Selector3/1 -> Bus to Vector/1  "<Navigation Message>"
  Bus to Vector1/1 -> Scope 1/1
  Bus to Vector2/1 -> Scope 3/1
  Bus Selector3/3 -> Bus to Vector2/1  "<Acoustic Message>"
  Bus Selector3/2 -> Bus to Vector1/1  "<Lidar Data Input>"
  Read/1 -> Scope 4/1

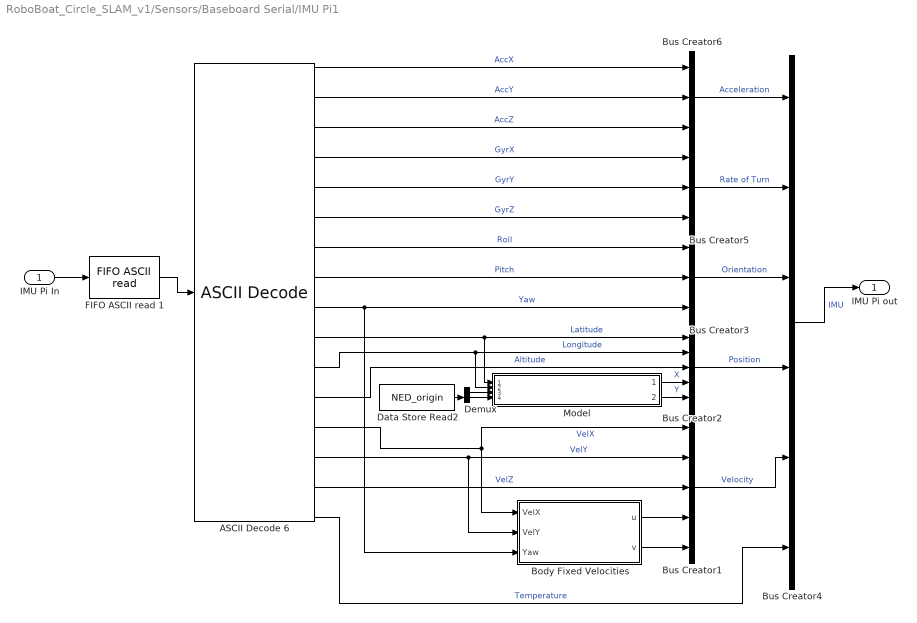
== system RoboBoat_Circle_SLAM_v1/Sensors/Baseboard Serial/IMU Pi1 ==
  IMU Pi In : Inport
  ASCII Decode 6 : xpcseriallib/ASCII Decode   format=AccX:%f AccY:%f AccZ:%f GyrX:%f GyrY:%f GyrZ:%f Roll:%f Pitch:%f Yaw:%f Lat:%f Long:%f Alt:%f VelX:%f VelY:%f VelZ:%f Temp:%f \r\n  nvars=16  vartypes={}
  Body Fixed Velocities : MATLAB Function  TreatAsAtomicUnit=on
  Bus Creator1 : BusCreator  Inputs=5
  Bus Creator2 : BusCreator  Inputs=5
  Bus Creator3 : BusCreator  Inputs=3
  Bus Creator4 : BusCreator  Inputs=6
  Bus Creator5 : BusCreator  Inputs=3
  Bus Creator6 : BusCreator  Inputs=3
  Data Store Read2 : DataStoreRead  DataStoreName=NED_origin
  Demux : Demux  Outputs=2
  FIFO ASCII read 1 : xpcseriallib/FIFO ASCII read   header={'AccX:'}  term=[13 10]  hold=Zero output if no new data  enable=off  maxsize=1024  outputtype=8 bit uint null terminated  sampletime=-1
  Model : ModelReference  ModelNameDialog=LLA2NEDv6.slx  SimulationMode=Normal  ModelReferenceVersion=1.2057  CopyOfModelName=LLA2NEDv6.slx  DefaultDataLogging=on
  IMU Pi out : Outport
  wires:
  IMU Pi In/1 -> FIFO ASCII read 1/1
  FIFO ASCII read 1/1 -> ASCII Decode 6/1
  Bus Creator4/1 -> IMU Pi out/1  "IMU"
  Data Store Read2/1 -> Demux/1
  Demux/1 -> Model/3
  Demux/2 -> Model/4
  Bus Creator1/1 -> Bus Creator4/5  "Velocity"
  Bus Creator2/1 -> Bus Creator4/4  "Position"
  Bus Creator3/1 -> Bus Creator4/3  "Orientation"
  Bus Creator5/1 -> Bus Creator4/2  "Rate of Turn"
  Bus Creator6/1 -> Bus Creator4/1  "Acceleration"
  ASCII Decode 6/1 -> Bus Creator6/1  "AccX"
  ASCII Decode 6/2 -> Bus Creator6/2  "AccY"
  ASCII Decode 6/3 -> Bus Creator6/3  "AccZ"
  ASCII Decode 6/4 -> Bus Creator5/1  "GyrX"
  ASCII Decode 6/5 -> Bus Creator5/2  "GyrY"
  ASCII Decode 6/6 -> Bus Creator5/3  "GyrZ"
  ASCII Decode 6/7 -> Bus Creator3/1  "Roll"
  ASCII Decode 6/8 -> Bus Creator3/2  "Pitch"
  ASCII Decode 6/9 -> Body Fixed Velocities/3(Yaw), Bus Creator3/3  "Yaw"
  ASCII Decode 6/10 -> Model/1, Bus Creator2/1  "Latitude"
  ASCII Decode 6/11 -> Model/2, Bus Creator2/2  "Longitude"
  ASCII Decode 6/12 -> Bus Creator2/3  "Altitude"
  Model/1 -> Bus Creator2/4  "X"
  Model/2 -> Bus Creator2/5  "Y"
  ASCII Decode 6/13 -> Bus Creator1/1, Body Fixed Velocities/1(VelX)  "VelX"
  ASCII Decode 6/14 -> Body Fixed Velocities/2(VelY), Bus Creator1/2  "VelY"
  ASCII Decode 6/15 -> Bus Creator1/3  "VelZ"
  Body Fixed Velocities/1(u) -> Bus Creator1/4
  Body Fixed Velocities/2(v) -> Bus Creator1/5
  ASCII Decode 6/16 -> Bus Creator4/6  "Temperature"

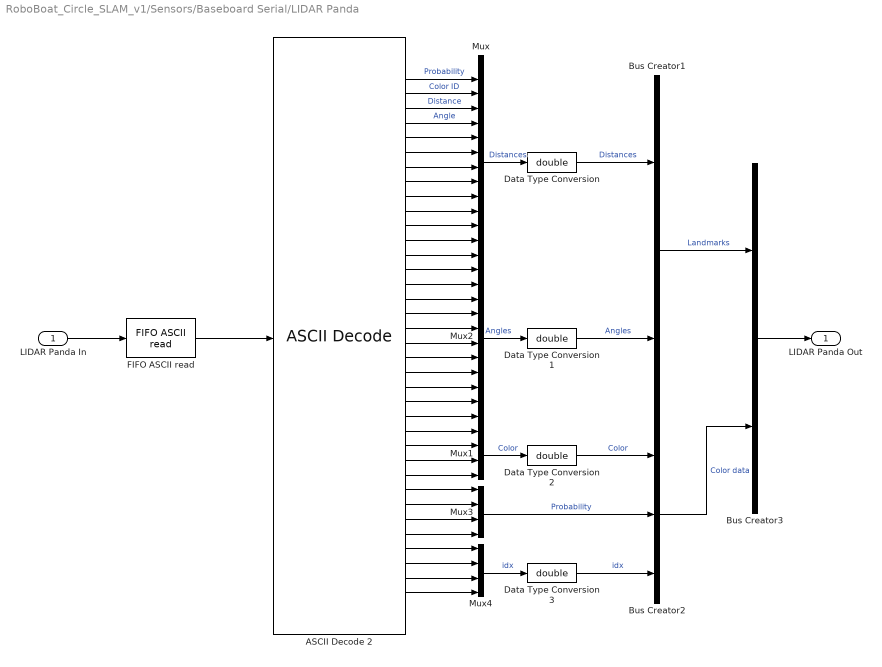
== system RoboBoat_Circle_SLAM_v1/Sensors/Baseboard Serial/LIDAR Panda ==
  LIDAR Panda In : Inport
  ASCII Decode 2 : xpcseriallib/ASCII Decode   format=A:%d B:%d C:%d D:%d E:%d F:%d G:%d H:%d I:%d J:%d K:%d L:%d M:%d N:%d O:%d P:%d Q:%d R:%d S:%d T:%d U:%d V:%d W:%d X:%d C1:%d C2:%d C3:%d C4:%d P1:%f P2:%f P3:%f P4:%f I1:%d I2:%d I3:%d I4:%d \r\n  nvars=36  vartypes={}
  Bus Creator1 : BusCreator  Inputs=2
  Bus Creator2 : BusCreator  Inputs=3
  Bus Creator3 : BusCreator  Inputs=2
  Data Type Conversion{,1..3} (4 alike) : DataTypeConversion  OutDataTypeStr=double
  "FIFO ASCII read " : xpcseriallib/FIFO ASCII read   header={'A:'}  term=[13 10]  hold=Zero output if no new data  enable=off  maxsize=1024  outputtype=8 bit uint null terminated  sampletime=-1
  Mux : Mux  Inputs=12
  Mux1 : Mux
  Mux2 : Mux  Inputs=12
  Mux3 : Mux
  Mux4 : Mux
  LIDAR Panda Out : Outport
  wires:
  LIDAR Panda In/1 -> "FIFO ASCII read "/1
  "FIFO ASCII read "/1 -> ASCII Decode 2/1
  ASCII Decode 2/3 -> Mux/3  "Distance"
  ASCII Decode 2/2 -> Mux/2  "Color ID"
  ASCII Decode 2/4 -> Mux/4  "Angle"
  ASCII Decode 2/1 -> Mux/1  "Probability"
  ASCII Decode 2/7 -> Mux/7
  ASCII Decode 2/10 -> Mux/10
  ASCII Decode 2/11 -> Mux/11
  ASCII Decode 2/6 -> Mux/6
  ASCII Decode 2/8 -> Mux/8
  ASCII Decode 2/9 -> Mux/9
  ASCII Decode 2/12 -> Mux/12
  ASCII Decode 2/5 -> Mux/5
  ASCII Decode 2/13 -> Mux2/1
  ASCII Decode 2/15 -> Mux2/3
  ASCII Decode 2/22 -> Mux2/10
  ASCII Decode 2/23 -> Mux2/11
  ASCII Decode 2/17 -> Mux2/5
  ASCII Decode 2/18 -> Mux2/6
  ASCII Decode 2/14 -> Mux2/2
  ASCII Decode 2/24 -> Mux2/12
  ASCII Decode 2/20 -> Mux2/8
  ASCII Decode 2/19 -> Mux2/7
  ASCII Decode 2/21 -> Mux2/9
  ASCII Decode 2/16 -> Mux2/4
  ASCII Decode 2/25 -> Mux1/1
  ASCII Decode 2/28 -> Mux1/4
  ASCII Decode 2/26 -> Mux1/2
  ASCII Decode 2/27 -> Mux1/3
  ASCII Decode 2/30 -> Mux3/2
  ASCII Decode 2/31 -> Mux3/3
  ASCII Decode 2/32 -> Mux3/4
  ASCII Decode 2/29 -> Mux3/1
  ASCII Decode 2/36 -> Mux4/4
  ASCII Decode 2/34 -> Mux4/2
  ASCII Decode 2/35 -> Mux4/3
  ASCII Decode 2/33 -> Mux4/1
  Mux/1 -> Data Type Conversion/1  "Distances"
  Mux2/1 -> Data Type Conversion1/1  "Angles"
  Mux1/1 -> Data Type Conversion2/1  "Color"
  Mux3/1 -> Bus Creator2/2  "Probability"
  Mux4/1 -> Data Type Conversion3/1  "idx"
  Bus Creator1/1 -> Bus Creator3/1  "Landmarks"
  Bus Creator2/1 -> Bus Creator3/2  "Color data"
  Bus Creator3/1 -> LIDAR Panda Out/1
  Data Type Conversion/1 -> Bus Creator1/1  "Distances"
  Data Type Conversion1/1 -> Bus Creator1/2  "Angles"
  Data Type Conversion2/1 -> Bus Creator2/1  "Color"
  Data Type Conversion3/1 -> Bus Creator2/3  "idx"

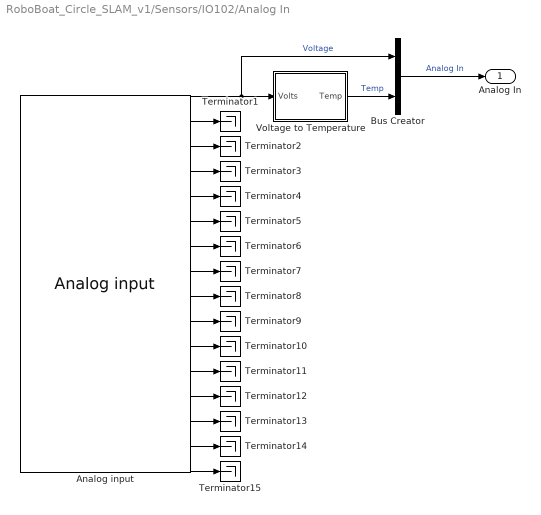
== system RoboBoat_Circle_SLAM_v1/Sensors/IO102/Analog In ==
  Analog input : speedgoatlib_IO102/Analog input  id=1  channels=[1,2,3,4,5,6,7,8,9,10,11,12,13,14,15,16]  range=2  high_voltage=off  adCoupling=1  ts=-1  pciSlot=-1
  Bus Creator : BusCreator  Inputs=2
  Terminator{1..15} (15 alike) : Terminator
  Voltage to Temperature : MATLAB Function  TreatAsAtomicUnit=on
  Analog In : Outport
  wires:
  Bus Creator/1 -> Analog In/1  "Analog In"
  Analog input/1 -> Bus Creator/1, Voltage to Temperature/1(Volts)  "Voltage"
  Voltage to Temperature/1(Temp) -> Bus Creator/2  "Temp"
  Analog input/2 -> Terminator1/1
  Analog input/3 -> Terminator2/1
  Analog input/4 -> Terminator3/1
  Analog input/5 -> Terminator4/1
  Analog input/6 -> Terminator5/1
  Analog input/7 -> Terminator6/1
  Analog input/8 -> Terminator7/1
  Analog input/9 -> Terminator8/1
  Analog input/10 -> Terminator9/1
  Analog input/11 -> Terminator10/1
  Analog input/12 -> Terminator11/1
  Analog input/13 -> Terminator12/1
  Analog input/14 -> Terminator13/1
  Analog input/15 -> Terminator14/1
  Analog input/16 -> Terminator15/1

== system RoboBoat_Circle_SLAM_v1/Sensors/IO102/Digital In ==
  Bus Creator : BusCreator  Inputs=1
  Digital input : speedgoatlib_IO102/Digital input  id=1  channels=[1,2,3,4,5,6,7,8]  ts=-1  pciSlot=-1
  Terminator{1,17..22} (7 alike) : Terminator
  Digital In : Outport
  wires:
  Bus Creator/1 -> Digital In/1  "Digital In"
  Digital input/8 -> Bus Creator/1  "Auto RC"
  Digital input/2 -> Terminator17/1
  Digital input/3 -> Terminator18/1
  Digital input/4 -> Terminator19/1
  Digital input/5 -> Terminator20/1
  Digital input/6 -> Terminator21/1
  Digital input/7 -> Terminator22/1
  Digital input/1 -> Terminator1/1

== matlab function RoboBoat_Circle_SLAM_v1/Sinks/MATLAB Function ==
  data: PortPow input; PortV output; StbdPow input; StbdV output
function [PortV, StbdV] = toVoltage(PortPow,StbdPow)
%Written By Anderson Lebbad on June 19, 2015
%Last Edited by:
%
%This function converts a desired value (0-100%, positive or negative) for
%each thruster to drive voltages.

%Signal is biased by 2.5 as it is voltage neutral, 5v control signal
PortV = -PortPow/100*2.5+2.5;
StbdV = StbdPow/100*2.5+2.5;

end

== matlab function RoboBoat_Circle_SLAM_v1/Sensors/Baseboard Serial/IMU Pi1/Body Fixed Velocities ==
  data: VelX input; u output; VelY input; Yaw input; v output
function [u,v] = VelNED2VelBF(VelX,VelY,Yaw)
%Written By Anderson Lebbad on June 22, 2015.
%Last Edited by:
%
%This functon converts NED velocities into the body fixed frame for system
%identification and use with models.

u = VelX*cos(Yaw*pi/180)+VelY*sin(Yaw*pi/180);
v = VelY*cos(Yaw*pi/180)-VelX*sin(Yaw*pi/180);

end

== matlab function RoboBoat_Circle_SLAM_v1/Sensors/IO102/Analog In/Voltage to Temperature ==
  data: Volts input; Temp output
function Temp = VtoC(Volts)
%Written By Anderson Lebbad on June 19, 2015
%Last Edited by:
%
%This function converts the voltage from the type E thermocouple to the
%equivalent temperature in degrees celsius

mV = -Volts*10^3;

T_0 = 250.146;
mV_0 = 17.191713;
p1 = 13.115522;
p2 = 1.1780364;
p3 = 0.036422433;
p4 = 0.00039584261;
q1 = 0.093112756;
q2 = 0.0029804232;
q3 = 0.000033263032;

Temp = T_0 + ((mV-mV_0)*(p1+(mV-mV_0)*(p2+(mV-mV_0)*(p3+p4*(mV-mV_0)))))/...
    (1+(mV-mV_0)*(q1+(mV-mV_0)*(q2+q3*(mV-mV_0))))

== matlab function RoboBoat_Circle_SLAM_v1/Sensors/1020 Comms/Data Update1 ==
  data: Valid input; ControlMode input; V output; C output; L output; A output; Data input; D1 output; D2 output; D3 output; D4 output; D5 output; D6 output; D7 output; D8 output; D9 output; D10 output; D11 output; D12 output; D13 output; D14 output; D15 output; D16 output; D17 output; D18 output; D19 output; D20 output; D21 output; D22 output; D23 output; D24 output; Activate input
function [V,C,L,A,D1,D2,D3,D4,D5,D6,D7,D8,D9,D10,D11,D12,D13,D14,D15,D16,D17,...
    D18,D19,D20,D21,D22,D23,D24] = dataSplit(Valid,ControlMode,Data,Activate)
%Written by Anderson Lebbad on August 10, 2014
%Last Edited by: Anderson Lebbad on September 11, 2014

%This function splits the data vector into the twelve channels it is
%composed of for communication

persistent HoldData

A = Activate;

if isempty(HoldData)
    HoldData = zeros(26,1);
end

L = 8;

if Valid == 1
    HoldData(1) = Valid;
    HoldData(2) = ControlMode;
    HoldData(3) = Data(1);
    HoldData(4) = Data(2);
    HoldData(5) = Data(3);
    HoldData(6) = Data(4);
    HoldData(7) = Data(5);
    HoldData(8) = Data(6);
    HoldData(9) = Data(7);
    HoldData(10) = Data(8);
    HoldData(11) = Data(9);
    HoldData(12) = Data(10);
    HoldData(13) = Data(11);
    HoldData(14) = Data(12);
    HoldData(15) = Data(13);
    HoldData(16) = Data(14);
    HoldData(17) = Data(15);
    HoldData(18) = Data(16);
    HoldData(19) = Data(17);
    HoldData(20) = Data(18);
    HoldData(21) = Data(19);
    HoldData(22) = Data(20);
    HoldData(23) = Data(21);
    HoldData(24) = Data(22);
    HoldData(25) = Data(23);
    HoldData(26) = Data(24);
end

V = HoldData(1);
C = HoldData(2);
D1 = HoldData(3);
D2 = HoldData(4);
D3 = HoldData(5);
D4 = HoldData(6);
D5 = HoldData(7);
D6 = HoldData(8);
D7 = HoldData(9);
D8 = HoldData(10);
D9 = HoldData(11);
D10 = HoldData(12);
D11 = HoldData(13);
D12 = HoldData(14);
D13 = HoldData(15);
D14 = HoldData(16);
D15 = HoldData(17);
D16 = HoldData(18);
D17 = HoldData(19);
D18 = HoldData(20);
D19 = HoldData(21);
D20 = HoldData(22);
D21 = HoldData(23);
D22 = HoldData(24);
D23 = HoldData(25);
D24 = HoldData(26);

end

== matlab function RoboBoat_Circle_SLAM_v1/Sensors/1020 Comms/Data Update2 ==
  data: Valid input; ControlMode input; V output; C output; L output; A output; Data input; D1 output; D2 output; D3 output; D4 output; D5 output; D6 output; D7 output; D8 output; D9 output; D10 output; D11 output; D12 output; D13 output; D14 output; D15 output; D16 output; D17 output; D18 output; D19 output; D20 output; D21 output; D22 output; D23 output; D24 output; Activate input
function [V,C,L,A,D1,D2,D3,D4,D5,D6,D7,D8,D9,D10,D11,D12,D13,D14,D15,D16,D17,...
    D18,D19,D20,D21,D22,D23,D24] = dataSplit(Valid,ControlMode,Data,Activate)
%Written by Anderson Lebbad on August 10, 2014
%Last Edited by: Anderson Lebbad on September 11, 2014

%This function splits the data vector into the twelve channels it is
%composed of for communication

persistent HoldData

if isempty(HoldData)
    HoldData = zeros(26,1);
    HoldData(2) = 2;
end

if Valid == 1
    HoldData(1) = Valid;
    HoldData(2) = ControlMode;
    HoldData(3) = Data(1);
    HoldData(4) = Data(2);
    HoldData(5) = Data(3);
    HoldData(6) = Data(4);
    HoldData(7) = Data(5);
    HoldData(8) = Data(6);
    HoldData(9) = Data(7);
    HoldData(10) = Data(8);
    HoldData(11) = Data(9);
    HoldData(12) = Data(10);
    HoldData(13) = Data(11);
    HoldData(14) = Data(12);
    HoldData(15) = Data(13);
    HoldData(16) = Data(14);
    HoldData(17) = Data(15);
    HoldData(18) = Data(16);
    HoldData(19) = Data(17);
    HoldData(20) = Data(18);
    HoldData(21) = Data(19);
    HoldData(22) = Data(20);
    HoldData(23) = Data(21);
    HoldData(24) = Data(22);
    HoldData(25) = Data(23);
    HoldData(26) = Data(24);
end

V = HoldData(1);
C = HoldData(2);
L = 8;
A = Activate;
D1 = HoldData(3);
D2 = HoldData(4);
D3 = HoldData(5);
D4 = HoldData(6);
D5 = HoldData(7);
D6 = HoldData(8);
D7 = HoldData(9);
D8 = HoldData(10);
D9 = HoldData(11);
D10 = HoldData(12);
D11 = HoldData(13);
D12 = HoldData(14);
D13 = HoldData(15);
D14 = HoldData(16);
D15 = HoldData(17);
D16 = HoldData(18);
D17 = HoldData(19);
D18 = HoldData(20);
D19 = HoldData(21);
D20 = HoldData(22);
D21 = HoldData(23);
D22 = HoldData(24);
D23 = HoldData(25);
D24 = HoldData(26);

end
